simulink subsystem "standardVehicle"  (R2020b)
settings: Solver=VariableStepAuto  StartTime=0.0  StopTime=10.0  RelTol=1e-3
undefined symbols (not defined in the file): Kbr, vehicleMass
libraries: autolibshared x4
(part 3 of 3)

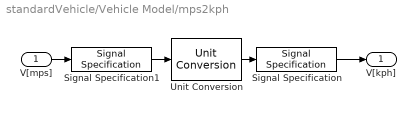
== system standardVehicle/Vehicle Model/mps2kph ==
  V[mps] : Inport
  Signal Specification : SignalSpecification  Unit=km/h
  Signal Specification1 : SignalSpecification  Unit=m/s
  Unit Conversion : UnitConversion
  V[kph] : Outport  VectorParamsAs1DForOutWhenUnconnected=off
  wires:
  V[mps]/1 -> Signal Specification1/1
  Unit Conversion/1 -> Signal Specification/1
  Signal Specification1/1 -> Unit Conversion/1
  Signal Specification/1 -> V[kph]/1
